simulink model "mmc"  (R2023b)
settings: Solver=VariableStepAuto  StartTime=0.0  StopTime=2  RelTol=1e-3
values from neighbouring files (symbols this model uses):
  ab0_to_cell = inv(cell_to_2ab0)    [init_mmc.m]
  cell_to_2ab0 = kron(abc_to_ab0, abc_to_ab0)    [init_mmc.m]
  grid_to_cell = kron(eye(3), ones(3, 1))    [init_mmc.m]
  J = [0 -1; 1 0]    [SafetyFilterSystemDPC.m]    (also in init_mmc.m)
  machine_to_cell = kron(ones(3, 1), eye(3))    [init_mmc.m]
  volt_to_cell = [      [          1 0 0 0 0 0 ... (first row only)    [init_mmc.m]
undefined symbols (not defined in the file or in its folder): cpu, ctrl, DiscIntNeverNeededParam, fdesignblkfcn, gcbh, grid, load1, machine, mmc, pq_ctrl, sim, soa
libraries: eeDiscretePi x9, spsabctodq0Lib x9, spsThreePhaseSeriesRLCBranchLib x8, dsparch4 x6, spsControlledVoltageSourceLib x6, spsThreePhaseVIMeasurementLib x6, eeGeneralControl x5, spsBreakerLib x3, spsGroundLib x3, library x3, spsThreePhaseBreakerLib x2, spsdq0toabcLib x2
(part 2 of 2)

== system mmc/CPU/abs ==
  in : Inport
  Complex to Magnitude-Angle1 : ComplexToMagnitudeAngle
  Demux : Demux  Outputs=2
  Real-Imag to Complex1 : RealImagToComplex
  Terminator : Terminator
  out : Outport
  wires:
  Complex to Magnitude-Angle1/1 -> out/1  "V_pcc_meas"
  Demux/2 -> Real-Imag to Complex1/2
  Demux/1 -> Real-Imag to Complex1/1
  Complex to Magnitude-Angle1/2 -> Terminator/1
  Real-Imag to Complex1/1 -> Complex to Magnitude-Angle1/1
  in/1 -> Demux/1

== system mmc/CPU/abs1 ==
  in : Inport
  Dot Product : DotProduct  OutDataTypeStr=Inherit: Inherit via internal rule
  Sqrt3 : Sqrt
  out : Outport
  wires:
  Sqrt3/1 -> out/1
  in/1 -> Dot Product/2, Dot Product/1
  Dot Product/1 -> Sqrt3/1

== system mmc/CPU/current controller (grid) ==
  u_ref : Inport
  u : Inport  Port=2
  antiwind : Inport  Port=3
  enable : Inport  Port=4
  Constant1 : Constant  Value=[0; 0]
  NOT1 : Logic  Operator=NOT  IconShape=distinctive  AllPortsSameDT=off  OutDataTypeStr=boolean
  PICtrl : eeDiscretePi/Discrete PI Controller  Kp=ctrl.grid.ictrl.kp  Ki=ctrl.grid.ictrl.ki  Kaw=100  x0=0  Ts=-1
      settings: LibrarySourceBlock=ee_sl_lib/General Control/Discrete PI Controller
  Sum : Sum  Inputs=|+-
  Switch : Switch  Criteria=u2 > Threshold  SaturateOnIntegerOverflow=off  InputSameDT=off
  y : Outport
  wires:
  u_ref/1 -> Sum/1
  u/1 -> Sum/2
  NOT1/1 -> Switch/2, PICtrl/3
  enable/1 -> NOT1/1
  PICtrl/1 -> y/1  "y"
  antiwind/1 -> PICtrl/2
  Sum/1 -> Switch/3
  Constant1/1 -> Switch/1
  Switch/1 -> PICtrl/1

== system mmc/CPU/dc voltage controller ==
  u_ref : Inport
  u : Inport  Port=2
  antiwind : Inport  Port=3
  enable : Inport  Port=4
  Constant1 : Constant  Value=zeros(1,1)
  NOT1 : Logic  Operator=NOT  IconShape=distinctive  AllPortsSameDT=off  OutDataTypeStr=boolean
  PICtrl : eeDiscretePi/Discrete PI Controller  Kp=ctrl.vdcctrl.kp  Ki=ctrl.vdcctrl.ki  Kaw=100  x0=0  Ts=-1
      settings: LibrarySourceBlock=ee_sl_lib/General Control/Discrete PI Controller
  Sum : Sum  Inputs=|+-
  Switch : Switch  Criteria=u2 > Threshold  SaturateOnIntegerOverflow=off  InputSameDT=off
  y : Outport
  wires:
  u_ref/1 -> Sum/1
  u/1 -> Sum/2
  NOT1/1 -> Switch/2, PICtrl/3
  enable/1 -> NOT1/1
  PICtrl/1 -> y/1  "y"
  antiwind/1 -> PICtrl/2
  Sum/1 -> Switch/3
  Constant1/1 -> Switch/1
  Switch/1 -> PICtrl/1

== system mmc/CPU/dc voltage controller1 ==
  u_ref : Inport
  u : Inport  Port=2
  antiwind : Inport  Port=3
  enable : Inport  Port=4
  Constant1 : Constant  Value=zeros(1,1)
  NOT1 : Logic  Operator=NOT  IconShape=distinctive  AllPortsSameDT=off  OutDataTypeStr=boolean
  PICtrl : eeDiscretePi/Discrete PI Controller  Kp=ctrl.vdcctrl.kp  Ki=ctrl.vdcctrl.ki/3  Kaw=100  x0=0  Ts=-1
      settings: LibrarySourceBlock=ee_sl_lib/General Control/Discrete PI Controller
  Sum : Sum  Inputs=|+-
  Switch : Switch  Criteria=u2 > Threshold  SaturateOnIntegerOverflow=off  InputSameDT=off
  y : Outport
  wires:
  u_ref/1 -> Sum/1
  u/1 -> Sum/2
  NOT1/1 -> Switch/2, PICtrl/3
  enable/1 -> NOT1/1
  PICtrl/1 -> y/1  "y"
  antiwind/1 -> PICtrl/2
  Sum/1 -> Switch/3
  Constant1/1 -> Switch/1
  Switch/1 -> PICtrl/1

== system mmc/CPU/dc voltage controller2 ==
  u_ref : Inport
  u : Inport  Port=2
  antiwind : Inport  Port=3
  enable : Inport  Port=4
  Constant1 : Constant  Value=zeros(1,1)
  NOT1 : Logic  Operator=NOT  IconShape=distinctive  AllPortsSameDT=off  OutDataTypeStr=boolean
  PICtrl : eeDiscretePi/Discrete PI Controller  Kp=ctrl.vdcctrl.kp  Ki=ctrl.vdcctrl.ki  Kaw=100  x0=0  Ts=-1
      settings: LibrarySourceBlock=ee_sl_lib/General Control/Discrete PI Controller
  Sum : Sum  Inputs=|+-
  Switch : Switch  Criteria=u2 > Threshold  SaturateOnIntegerOverflow=off  InputSameDT=off
  y : Outport
  wires:
  u_ref/1 -> Sum/1
  u/1 -> Sum/2
  NOT1/1 -> Switch/2, PICtrl/3
  enable/1 -> NOT1/1
  PICtrl/1 -> y/1  "y"
  antiwind/1 -> PICtrl/2
  Sum/1 -> Switch/3
  Constant1/1 -> Switch/1
  Switch/1 -> PICtrl/1

== system mmc/Measurements grid/BP100 ==
  In : Inport
  Generated Filter Block : dsparch4/Biquad Filter  Tag=BlockMethodSubSystem  FilterSource=Dialog parameters  CoeffSource=Specify via dialog  FilterObject=BQF  IIRFiltStruct=Direct form II  BiQuadCoeffs=[2 0 -2 1 -1.99993786796251327 0.999938262487757412]  ScaleValues=[1.99433834389553329e-07;77.3909708347894423]  IC=0  ICnum=0  ICden=0  a0Flag=Warning  optimizeScaleValues=off  ScaleValueMode=Specify via input port (g)  roundingMode=Floor  overflowMode=off  scaleValueFracLength=14  denProdOutputFracLength=30  denAccumFracLength=30  secondMemoryFracLength=15
  Out : Outport  VectorParamsAs1DForOutWhenUnconnected=off
  wires:
  In/1 -> Generated Filter Block/1
  Generated Filter Block/1 -> Out/1

== system mmc/Measurements grid/BP50_10 ==
  In : Inport
  Generated Filter Block : dsparch4/Biquad Filter  Tag=BlockMethodSubSystem  FilterSource=Dialog parameters  CoeffSource=Specify via dialog  FilterObject=BQF  IIRFiltStruct=Direct form II  BiQuadCoeffs=[2 0 -2 1 -1.99996903213533184 0.99996913076816718]  ScaleValues=[4.98592317955378183e-08;154.7819266430281]  IC=0  ICnum=0  ICden=0  a0Flag=Warning  optimizeScaleValues=off  ScaleValueMode=Specify via input port (g)  roundingMode=Floor  overflowMode=off  scaleValueFracLength=14  denProdOutputFracLength=30  denAccumFracLength=30  secondMemoryFracLength=15
  Out : Outport  VectorParamsAs1DForOutWhenUnconnected=off
  wires:
  In/1 -> Generated Filter Block/1
  Generated Filter Block/1 -> Out/1

== system mmc/Measurements grid/BP50_3 ==
  In : Inport
  Generated Filter Block : dsparch4/Biquad Filter  Tag=BlockMethodSubSystem  FilterSource=Dialog parameters  CoeffSource=Specify via dialog  FilterObject=BQF  IIRFiltStruct=Direct form II  BiQuadCoeffs=[2 0 -2 1 -1.99996903213533184 0.99996913076816718]  ScaleValues=[4.98592317955378183e-08;154.7819266430281]  IC=0  ICnum=0  ICden=0  a0Flag=Warning  optimizeScaleValues=off  ScaleValueMode=Specify via input port (g)  roundingMode=Floor  overflowMode=off  scaleValueFracLength=14  denProdOutputFracLength=30  denAccumFracLength=30  secondMemoryFracLength=15
  Out : Outport  VectorParamsAs1DForOutWhenUnconnected=off
  wires:
  In/1 -> Generated Filter Block/1
  Generated Filter Block/1 -> Out/1

== system mmc/Measurements machine/BP16_i ==
  In : Inport
  Generated Filter Block : dsparch4/Biquad Filter  Tag=BlockMethodSubSystem  FilterSource=Dialog parameters  CoeffSource=Specify via dialog  FilterObject=BQF  IIRFiltStruct=Direct form II  BiQuadCoeffs=[2 0 -2 1 -1.99998969920097514 0.999989710160291256]  ScaleValues=[1.09593161212728774e-08;234.728143507018871]  IC=0  ICnum=0  ICden=0  a0Flag=Warning  optimizeScaleValues=off  ScaleValueMode=Specify via input port (g)  roundingMode=Floor  overflowMode=off  scaleValueFracLength=14  denProdOutputFracLength=30  denAccumFracLength=30  secondMemoryFracLength=15
  Out : Outport  VectorParamsAs1DForOutWhenUnconnected=off
  wires:
  In/1 -> Generated Filter Block/1
  Generated Filter Block/1 -> Out/1

== system mmc/Measurements machine/BP16_v ==
  In : Inport
  Generated Filter Block : dsparch4/Biquad Filter  Tag=BlockMethodSubSystem  FilterSource=Dialog parameters  CoeffSource=Specify via dialog  FilterObject=BQF  IIRFiltStruct=Direct form II  BiQuadCoeffs=[2 0 -2 1 -1.99998969920097514 0.999989710160291256]  ScaleValues=[1.09593161212728774e-08;234.728143507018871]  IC=0  ICnum=0  ICden=0  a0Flag=Warning  optimizeScaleValues=off  ScaleValueMode=Specify via input port (g)  roundingMode=Floor  overflowMode=off  scaleValueFracLength=14  denProdOutputFracLength=30  denAccumFracLength=30  secondMemoryFracLength=15
  Out : Outport  VectorParamsAs1DForOutWhenUnconnected=off
  wires:
  In/1 -> Generated Filter Block/1
  Generated Filter Block/1 -> Out/1

== system mmc/dq_to_ab_g/Subsystem ==
  dq : Inport  PortDimensions=2
  wt : Inport  Port=2  PortDimensions=1
  Fcn : Fcn  Expr=u[1]*cos(u[3]) - u[2]*sin(u[3])
  Fcn1 : Fcn  Expr=u[1]*sin(u[3]) + u[2]*cos(u[3])
  Mux11 : Mux  Inputs=2
  Mux12 : Mux  Inputs=[2 1]
  Mux13 : Mux  Inputs=[2 1]
  alpha_beta : Outport  InitialOutput=[0,0]  VectorParamsAs1DForOutWhenUnconnected=off
  wires:
  wt/1 -> Mux13/2, Mux12/2
  Fcn1/1 -> Mux11/2
  Mux11/1 -> alpha_beta/1
  dq/1 -> Mux13/1, Mux12/1
  Fcn/1 -> Mux11/1
  Mux12/1 -> Fcn/1
  Mux13/1 -> Fcn1/1

== system mmc/dq_to_ab_g/Subsystem1 ==
  dq : Inport  PortDimensions=2
  wt : Inport  Port=2  PortDimensions=1
  Fcn : Fcn  Expr=u[1]*cos(u[3]) - u[2]*sin(u[3])
  Fcn1 : Fcn  Expr=u[1]*sin(u[3]) + u[2]*cos(u[3])
  Mux11 : Mux  Inputs=2
  Mux12 : Mux  Inputs=[2 1]
  Mux13 : Mux  Inputs=[2 1]
  alpha_beta : Outport  InitialOutput=[0,0]  VectorParamsAs1DForOutWhenUnconnected=off
  wires:
  wt/1 -> Mux13/2, Mux12/2
  Fcn1/1 -> Mux11/2
  Mux11/1 -> alpha_beta/1
  dq/1 -> Mux13/1, Mux12/1
  Fcn/1 -> Mux11/1
  Mux12/1 -> Fcn/1
  Mux13/1 -> Fcn1/1

== system mmc/dq_to_ab_m/Subsystem ==
  dq : Inport  PortDimensions=2
  wt : Inport  Port=2  PortDimensions=1
  Fcn : Fcn  Expr=u[1]*cos(u[3]) - u[2]*sin(u[3])
  Fcn1 : Fcn  Expr=u[1]*sin(u[3]) + u[2]*cos(u[3])
  Mux11 : Mux  Inputs=2
  Mux12 : Mux  Inputs=[2 1]
  Mux13 : Mux  Inputs=[2 1]
  alpha_beta : Outport  InitialOutput=[0,0]  VectorParamsAs1DForOutWhenUnconnected=off
  wires:
  wt/1 -> Mux13/2, Mux12/2
  Fcn1/1 -> Mux11/2
  Mux11/1 -> alpha_beta/1
  dq/1 -> Mux13/1, Mux12/1
  Fcn/1 -> Mux11/1
  Mux12/1 -> Fcn/1
  Mux13/1 -> Fcn1/1

== system mmc/dq_to_ab_m/Subsystem1 ==
  dq : Inport  PortDimensions=2
  wt : Inport  Port=2  PortDimensions=1
  Fcn : Fcn  Expr=u[1]*cos(u[3]) - u[2]*sin(u[3])
  Fcn1 : Fcn  Expr=u[1]*sin(u[3]) + u[2]*cos(u[3])
  Mux11 : Mux  Inputs=2
  Mux12 : Mux  Inputs=[2 1]
  Mux13 : Mux  Inputs=[2 1]
  alpha_beta : Outport  InitialOutput=[0,0]  VectorParamsAs1DForOutWhenUnconnected=off
  wires:
  wt/1 -> Mux13/2, Mux12/2
  Fcn1/1 -> Mux11/2
  Mux11/1 -> alpha_beta/1
  dq/1 -> Mux13/1, Mux12/1
  Fcn/1 -> Mux11/1
  Mux12/1 -> Fcn/1
  Mux13/1 -> Fcn1/1

== system mmc/dq_to_ab_ns/Subsystem ==
  dq : Inport  PortDimensions=2
  wt : Inport  Port=2  PortDimensions=1
  Fcn : Fcn  Expr=u[1]*cos(u[3]) - u[2]*sin(u[3])
  Fcn1 : Fcn  Expr=u[1]*sin(u[3]) + u[2]*cos(u[3])
  Mux11 : Mux  Inputs=2
  Mux12 : Mux  Inputs=[2 1]
  Mux13 : Mux  Inputs=[2 1]
  alpha_beta : Outport  InitialOutput=[0,0]  VectorParamsAs1DForOutWhenUnconnected=off
  wires:
  wt/1 -> Mux13/2, Mux12/2
  Fcn1/1 -> Mux11/2
  Mux11/1 -> alpha_beta/1
  dq/1 -> Mux13/1, Mux12/1
  Fcn/1 -> Mux11/1
  Mux12/1 -> Fcn/1
  Mux13/1 -> Fcn1/1

== system mmc/dq_to_ab_ns/Subsystem1 ==
  dq : Inport  PortDimensions=2
  wt : Inport  Port=2  PortDimensions=1
  Fcn : Fcn  Expr=u[1]*cos(u[3]) - u[2]*sin(u[3])
  Fcn1 : Fcn  Expr=u[1]*sin(u[3]) + u[2]*cos(u[3])
  Mux11 : Mux  Inputs=2
  Mux12 : Mux  Inputs=[2 1]
  Mux13 : Mux  Inputs=[2 1]
  alpha_beta : Outport  InitialOutput=[0,0]  VectorParamsAs1DForOutWhenUnconnected=off
  wires:
  wt/1 -> Mux13/2, Mux12/2
  Fcn1/1 -> Mux11/2
  Mux11/1 -> alpha_beta/1
  dq/1 -> Mux13/1, Mux12/1
  Fcn/1 -> Mux11/1
  Mux12/1 -> Fcn/1
  Mux13/1 -> Fcn1/1

== system mmc/CPU/PQ Ctrl/PQ Calc ==
  v_pcc_dq : Inport
  i_bp_dq : Inport  Port=2
  Gain2 : Gain  Gain=J  Multiplication=Matrix(K*u) (u vector)
  Low-Pass Filter (Discrete or Continuous) : eeGeneralControl/Low-Pass Filter (Discrete or Continuous)  K=1  T=1/machine.w  B=inf  A=-inf  init_option=Inherited from block input  x0=0  Ts=-1
  Mux : Mux  Inputs=2
  Product1 : Product  Multiplication=Matrix(*)
  Product2 : Product  Multiplication=Matrix(*)
  Transpose : Math  Operator=transpose
  Transpose1 : Math  Operator=transpose
  PQ : Outport
  wires:
  Gain2/1 -> Transpose1/1
  v_pcc_dq/1 -> Transpose/1, Gain2/1
  i_bp_dq/1 -> Product1/2, Product2/2
  Product1/1 -> Mux/1
  Product2/1 -> Mux/2
  Transpose1/1 -> Product2/1
  Transpose/1 -> Product1/1
  Low-Pass Filter (Discrete or Continuous)/1 -> PQ/1
  Mux/1 -> Low-Pass Filter (Discrete or Continuous)/1

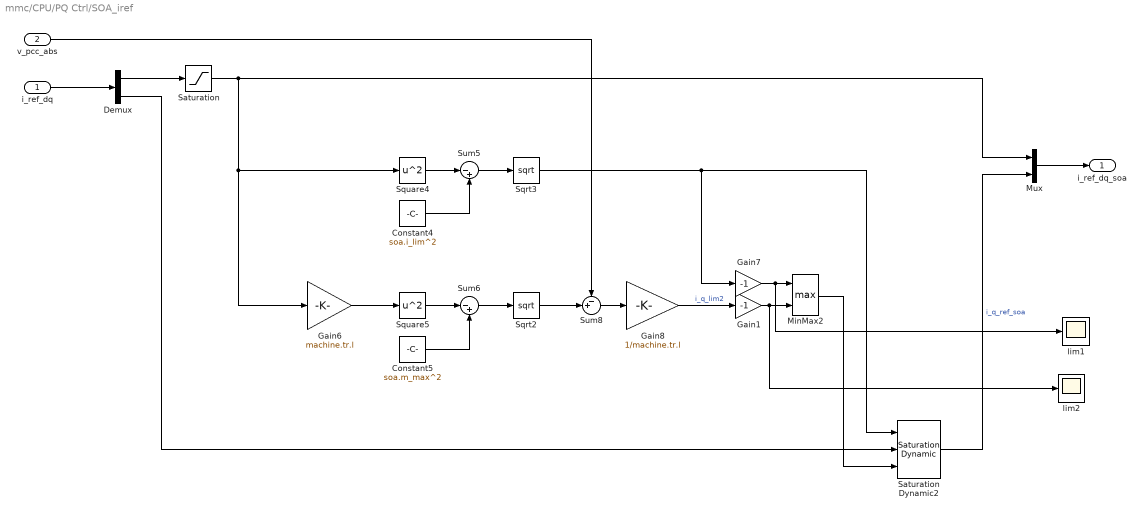
== system mmc/CPU/PQ Ctrl/SOA_iref ==
  i_ref_dq : Inport
  v_pcc_abs : Inport  Port=2
  Constant4 : Constant  Value=soa.i_lim^2
  Constant5 : Constant  Value=soa.m_max^2
  Demux : Demux  Outputs=2
  Gain1 : Gain  Gain=-1
  Gain6 : Gain  Gain=machine.tr.l
  Gain7 : Gain  Gain=-1
  Gain8 : Gain  Gain=1/machine.tr.l
  MinMax2 : MinMax  Function=max  Inputs=2
  Mux : Mux  Inputs=2
  Saturation : Saturate  UpperLimit=soa.i_lim  LowerLimit=-soa.i_lim
  Saturation Dynamic2 : simulink/Discontinuities/Saturation Dynamic  OutMin=[]  OutMax=[]  OutDataTypeStr=Inherit: Same as second input  OutDataType=fixdt(1, 16)  OutScaling=2^-10  DoSatur=off
  Sqrt2 : Sqrt
  Sqrt3 : Sqrt
  Square4 : Math  Operator=square
  Square5 : Math  Operator=square
  Sum5 : Sum  Inputs=|-+
  Sum6 : Sum  Inputs=|-+
  Sum8 : Sum  Inputs=-+|
  lim1 : Scope
  lim2 : Scope
  i_ref_dq_soa : Outport
  wires:
  Saturation/1 -> Square4/1, Gain6/1, Mux/1
  Gain8/1 -> Gain1/1  "i_q_lim2"
  Sqrt3/1 -> Saturation Dynamic2/1, Gain7/1
  Gain6/1 -> Square5/1
  Demux/1 -> Saturation/1
  Square4/1 -> Sum5/1
  Sqrt2/1 -> Sum8/2
  Square5/1 -> Sum6/1
  Sum8/1 -> Gain8/1
  Constant5/1 -> Sum6/2
  Sum5/1 -> Sqrt3/1
  Demux/2 -> Saturation Dynamic2/2
  Constant4/1 -> Sum5/2
  MinMax2/1 -> Saturation Dynamic2/3
  i_ref_dq/1 -> Demux/1
  Gain7/1 -> lim1/1, MinMax2/1
  v_pcc_abs/1 -> Sum8/1
  Sum6/1 -> Sqrt2/1
  Saturation Dynamic2/1 -> Mux/2  "i_q_ref_soa"
  Mux/1 -> i_ref_dq_soa/1
  Gain1/1 -> lim2/1, MinMax2/2

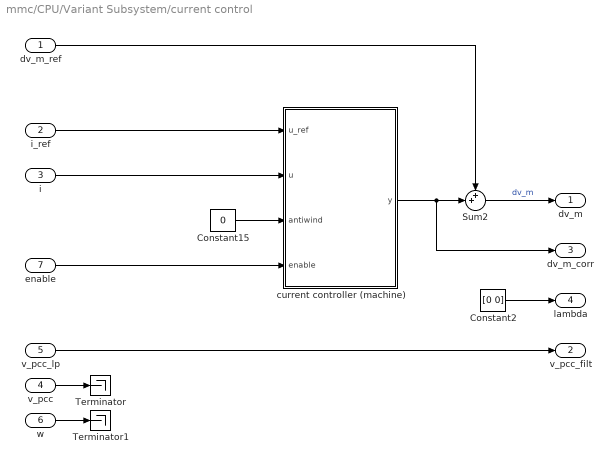
== system mmc/CPU/Variant Subsystem/current control ==
  dv_m_ref : Inport
  i_ref : Inport  Port=2
  i : Inport  Port=3
  v_pcc : Inport  Port=4
  v_pcc_lp : Inport  Port=5
  w : Inport  Port=6
  enable : Inport  Port=7
  Constant15 : Constant  Value=0
  Constant2 : Constant  Value=[0 0]
  Sum2 : Sum  Inputs=++|
  Terminator : Terminator
  Terminator1 : Terminator
  current controller (machine) : Subsystem  VariantControl=overcurr_ctrl.sel==1
  dv_m : Outport
  v_pcc_filt : Outport  Port=2
  dv_m_corr : Outport  Port=3
  lambda : Outport  Port=4
  wires:
  i/1 -> current controller (machine)/2(u)
  Constant15/1 -> current controller (machine)/3(antiwind)
  dv_m_ref/1 -> Sum2/1
  enable/1 -> current controller (machine)/4(enable)
  v_pcc/1 -> Terminator/1
  Sum2/1 -> dv_m/1  "dv_m"
  i_ref/1 -> current controller (machine)/1(u_ref)
  w/1 -> Terminator1/1
  current controller (machine)/1(y) -> dv_m_corr/1, Sum2/2
  Constant2/1 -> lambda/1
  v_pcc_lp/1 -> v_pcc_filt/1

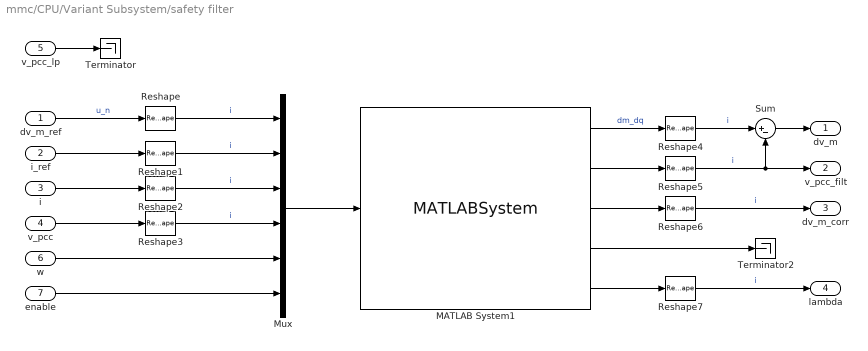
== system mmc/CPU/Variant Subsystem/safety filter ==
  dv_m_ref : Inport
  i_ref : Inport  Port=2
  i : Inport  Port=3
  v_pcc : Inport  Port=4
  v_pcc_lp : Inport  Port=5
  w : Inport  Port=6
  enable : Inport  Port=7
  MATLAB System1 : MATLABSystem  System=SafetyFilterSystemDPC  ts=cpu.ts  f_data=safety.f_data  G_data=safety.G_data  V_data=safety.V_data  B_data=safety.B_data  nV_data=safety.nV_data  nB_data=safety.nB_data  gamma_V_data=safety.gamma_V_data  gamma_B_data=safety.gamma_B_data  r=machine.tr.r  l=machine.tr.l  init_vpcc_f=[1; 0]  SimulateUsing=Code generation
      mask Type: SafetyFilterSystemDPC
      mask Display:
      | disp('SafetyFilterSystemDPC');
      | port_label('input',1,'u');
      | port_label('output',1,'m');
      | port_label('output',2,'v_pcc_f');
      | port_label('output',3,'dm_corr');
      | port_label('output',4,'active');
      | port_label('output',5,'lambda');
  Mux : Mux  Inputs=[2 2 2 2 1 1]
  Reshape{,1..3} (4 alike) : Reshape  OutputDimensionality=Customize  OutputDimensions=[2,1]
  Reshape{4..7} (4 alike) : Reshape  OutputDimensionality=Customize  OutputDimensions=[2]
  Sum : Sum  Inputs=|+-
  Terminator : Terminator
  Terminator2 : Terminator
  dv_m : Outport
  v_pcc_filt : Outport  Port=2
  dv_m_corr : Outport  Port=3
  lambda : Outport  Port=4
  wires:
  Reshape5/1 -> Sum/2, v_pcc_filt/1  "i"
  Reshape1/1 -> Mux/2  "i"
  Reshape6/1 -> dv_m_corr/1  "i"
  enable/1 -> Mux/6
  Reshape7/1 -> lambda/1  "i"
  MATLAB System1/3 -> Reshape6/1
  v_pcc/1 -> Reshape3/1
  MATLAB System1/2 -> Reshape5/1
  w/1 -> Mux/5
  MATLAB System1/5 -> Reshape7/1
  MATLAB System1/1 -> Reshape4/1  "dm_dq"
  Reshape2/1 -> Mux/3  "i"
  dv_m_ref/1 -> Reshape/1  "u_n"
  Reshape/1 -> Mux/1  "i"
  i/1 -> Reshape2/1
  i_ref/1 -> Reshape1/1
  Reshape3/1 -> Mux/4  "i"
  Mux/1 -> MATLAB System1/1
  MATLAB System1/4 -> Terminator2/1
  Sum/1 -> dv_m/1
  Reshape4/1 -> Sum/1  "i"
  v_pcc_lp/1 -> Terminator/1

== system mmc/CPU/Variant Subsystem/current control/current controller (machine) ==
  u_ref : Inport
  u : Inport  Port=2
  antiwind : Inport  Port=3
  enable : Inport  Port=4
  Constant1 : Constant  Value=[0; 0]
  NOT1 : Logic  Operator=NOT  IconShape=distinctive  AllPortsSameDT=off  OutDataTypeStr=boolean
  PICtrl : eeDiscretePi/Discrete PI Controller  Kp=ctrl.machine.ictrl.kp  Ki=ctrl.machine.ictrl.ki  Kaw=100  x0=0  Ts=-1
      settings: LibrarySourceBlock=ee_sl_lib/General Control/Discrete PI Controller
  Sum : Sum  Inputs=|+-
  Switch : Switch  Criteria=u2 > Threshold  SaturateOnIntegerOverflow=off  InputSameDT=off
  y : Outport
  wires:
  u_ref/1 -> Sum/1
  u/1 -> Sum/2
  NOT1/1 -> Switch/2, PICtrl/3
  enable/1 -> NOT1/1
  PICtrl/1 -> y/1  "y"
  antiwind/1 -> PICtrl/2
  Sum/1 -> Switch/3
  Constant1/1 -> Switch/1
  Switch/1 -> PICtrl/1
